simulink model "DynamicModelComplete"  (R2022b)
settings: configuration reference "WheelSimConfiguration" (kept outside this file)
settings Model: Creator=At  LastModifiedBy=MOSA
settings ConfigSetRef: SourceName=WheelSimConfiguration  SourceLocation=Base Workspace

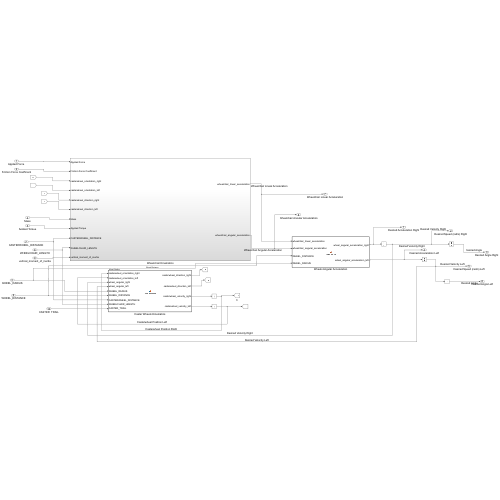
[thumbnail: Simulink's stored preview of the top-level diagram]
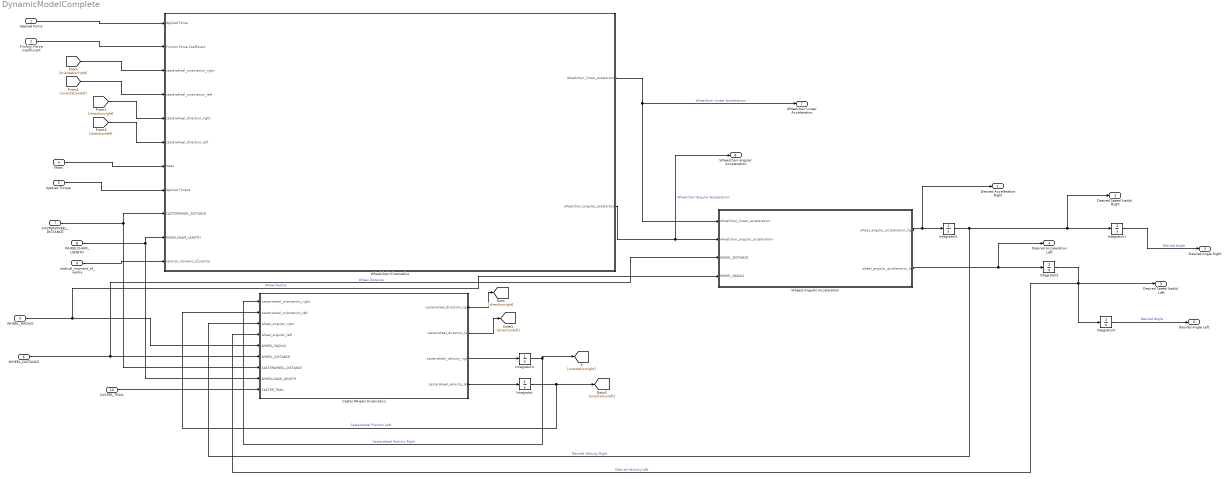
== system DynamicModelComplete ==
  "Applied Force " : Inport
  Friction Force Coefficient : Inport  Port=2
  WHEEL_RADIUS : Inport  Port=3
  Mass : Inport  Port=4
  Applied Torque : Inport  Port=5
  WHEEL_DISTANCE : Inport  Port=6
  CASTERWHEEL_DISTANCE : Inport  Port=7
  WHEELCHAIR_LENGTH : Inport  Port=8
  vertical_moment_of_inertia : Inport  Port=9
  CASTER_TRAIL : Inport  Port=10
  Caster Wheels Kinematics : MATLAB Function  TreatAsAtomicUnit=on
  Integrator{,1..5} (6 alike) : Integrator
  Wheelchair Kinematics : Subsystem
  Wheels Angular Acceleration : MATLAB Function  TreatAsAtomicUnit=on
  Desired Acceleration Right : Outport
  Desired Speed (rad/s) Right : Outport  Port=2
  Desired Angle Right : Outport  Port=3
  Desired Acceleration Left : Outport  Port=4
  Desired Speed (rad/s) Left : Outport  Port=5
  Desired Angle Left : Outport  Port=6
  Wheelchair Linear Acceleration : Outport  Port=7
  Wheelchair Angular Acceleration : Outport  Port=8
  wires:
  Integrator5/1 -> Caster Wheels Kinematics/3(wheel_angular_right), Integrator1/1, Desired Speed (rad/s) Right/1  "Desired Velocity Right"
  Integrator1/1 -> Desired Angle Right/1  "Desired Angle"
  Integrator2/1 -> Caster Wheels Kinematics/4(wheel_angular_left), Desired Speed (rad/s) Left/1, Integrator3/1  "Desired Velocity Left"
  Integrator3/1 -> Desired Angle Left/1  "Desired Angle"
  Wheels Angular Acceleration/1(wheel_angular_acceleration_right) -> Desired Acceleration Right/1, Integrator5/1
  Wheelchair Kinematics/1(wheelchair_linear_acceleration) -> Wheels Angular Acceleration/1(wheelchair_linear_acceleration), Wheelchair Linear Acceleration/1  "Wheelchair Linear Acceleration"
  Wheelchair Kinematics/2(wheelchair_angular_acceleration) -> Wheelchair Angular Acceleration/1, Wheels Angular Acceleration/2(wheelchair_angular_acceleration)  "Wheelchair Angular Acceleration"
  CASTERWHEEL_DISTANCE/1 -> Caster Wheels Kinematics/7(CASTERWHEEL_DISTANCE), Wheelchair Kinematics/9(CASTERWHEEL_DISTANCE)
  WHEELCHAIR_LENGTH/1 -> Caster Wheels Kinematics/8(WHEELCHAIR_LENGTH), Wheelchair Kinematics/10(WHEELCHAIR_LENGTH)
  vertical_moment_of_inertia/1 -> Wheelchair Kinematics/11(vertical_moment_of_inertia)
  "Applied Force "/1 -> Wheelchair Kinematics/1("Applied Force ")
  Friction Force Coefficient/1 -> Wheelchair Kinematics/2(Friction Force Coefficient)
  Mass/1 -> Wheelchair Kinematics/7(Mass)
  Applied Torque/1 -> Wheelchair Kinematics/8(Applied Torque)
  Caster Wheels Kinematics/3(casterwheel_velocity_right) -> Integrator4/1
  Caster Wheels Kinematics/4(casterwheel_velocity_left) -> Integrator/1
  Caster Wheels Kinematics/1(casterwheel_direction_right) -> [directionright]
  Integrator/1 -> [orientationleft], Caster Wheels Kinematics/2(casterwheel_orientation_left)  "Casterwheel Position Left"
  Integrator4/1 -> [orientationright], Caster Wheels Kinematics/1(casterwheel_orientation_right)  "Casterwheel Position Right"
  Caster Wheels Kinematics/2(casterwheel_direction_left) -> [directionleft]
  [directionleft] -> Wheelchair Kinematics/6(casterwheel_direction_left)
  [directionright] -> Wheelchair Kinematics/5(casterwheel_direction_right)
  [orientationleft] -> Wheelchair Kinematics/4(casterwheel_orientation_left)
  [orientationright] -> Wheelchair Kinematics/3(casterwheel_orientation_right)
  Wheels Angular Acceleration/2(wheel_angular_acceleration_left) -> Desired Acceleration Left/1, Integrator2/1
  CASTER_TRAIL/1 -> Caster Wheels Kinematics/9(CASTER_TRAIL)
  WHEEL_RADIUS/1 -> Wheels Angular Acceleration/4(WHEEL_RADIUS), Caster Wheels Kinematics/5(WHEEL_RADIUS)  "Wheel Radius"
  WHEEL_DISTANCE/1 -> Wheels Angular Acceleration/3(WHEEL_DISTANCE), Caster Wheels Kinematics/6(WHEEL_DISTANCE)  "Wheel Distance"

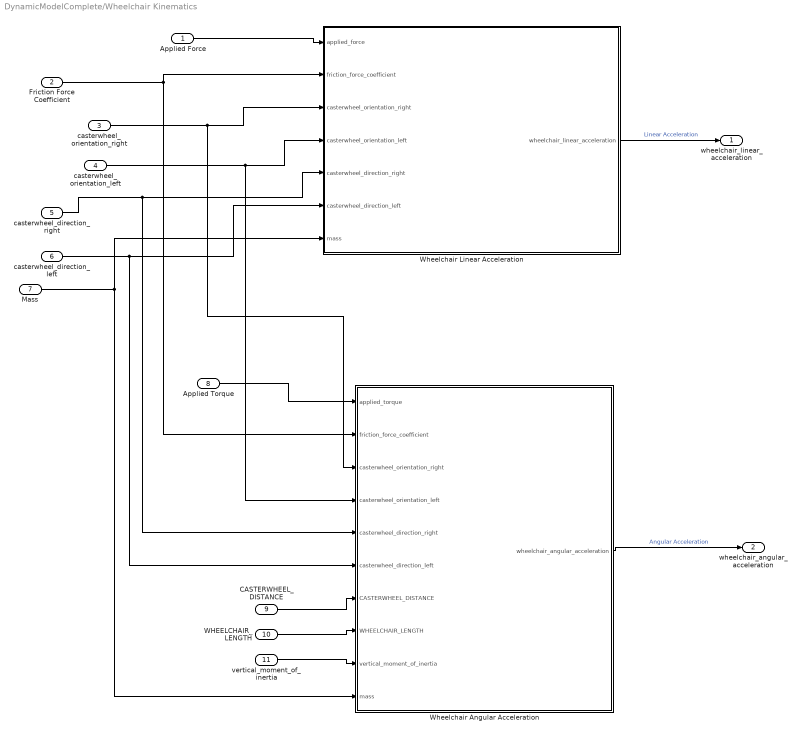
== system DynamicModelComplete/Wheelchair Kinematics ==
  "Applied Force " : Inport
  Friction Force Coefficient : Inport  Port=2
  casterwheel_orientation_right : Inport  Port=3
  casterwheel_orientation_left : Inport  Port=4
  casterwheel_direction_right : Inport  Port=5
  casterwheel_direction_left : Inport  Port=6
  Mass : Inport  Port=7
  Applied Torque : Inport  Port=8
  CASTERWHEEL_DISTANCE : Inport  Port=9
  WHEELCHAIR_LENGTH : Inport  Port=10
  vertical_moment_of_inertia : Inport  Port=11
  Wheelchair Angular Acceleration : MATLAB Function  TreatAsAtomicUnit=on
  Wheelchair Linear Acceleration : MATLAB Function  TreatAsAtomicUnit=on
  wheelchair_linear_acceleration : Outport
  wheelchair_angular_acceleration : Outport  Port=2
  wires:
  "Applied Force "/1 -> Wheelchair Linear Acceleration/1(applied_force)
  Mass/1 -> Wheelchair Angular Acceleration/10(mass), Wheelchair Linear Acceleration/7(mass)
  Applied Torque/1 -> Wheelchair Angular Acceleration/1(applied_torque)
  Wheelchair Linear Acceleration/1(wheelchair_linear_acceleration) -> wheelchair_linear_acceleration/1  "Linear Acceleration"
  Wheelchair Angular Acceleration/1(wheelchair_angular_acceleration) -> wheelchair_angular_acceleration/1  "Angular Acceleration"
  Friction Force Coefficient/1 -> Wheelchair Angular Acceleration/2(friction_force_coefficient), Wheelchair Linear Acceleration/2(friction_force_coefficient)
  casterwheel_orientation_right/1 -> Wheelchair Angular Acceleration/3(casterwheel_orientation_right), Wheelchair Linear Acceleration/3(casterwheel_orientation_right)
  casterwheel_orientation_left/1 -> Wheelchair Angular Acceleration/4(casterwheel_orientation_left), Wheelchair Linear Acceleration/4(casterwheel_orientation_left)
  casterwheel_direction_right/1 -> Wheelchair Angular Acceleration/5(casterwheel_direction_right), Wheelchair Linear Acceleration/5(casterwheel_direction_right)
  casterwheel_direction_left/1 -> Wheelchair Angular Acceleration/6(casterwheel_direction_left), Wheelchair Linear Acceleration/6(casterwheel_direction_left)
  CASTERWHEEL_DISTANCE/1 -> Wheelchair Angular Acceleration/7(CASTERWHEEL_DISTANCE)
  WHEELCHAIR_LENGTH/1 -> Wheelchair Angular Acceleration/8(WHEELCHAIR_LENGTH)
  vertical_moment_of_inertia/1 -> Wheelchair Angular Acceleration/9(vertical_moment_of_inertia)

== matlab function DynamicModelComplete/Wheelchair Kinematics/Wheelchair Angular Acceleration ==
  data: applied_torque input; friction_force_coefficient input; casterwheel_orientation_right input; casterwheel_orientation_left input; casterwheel_direction_right input; casterwheel_direction_left input; CASTERWHEEL_DISTANCE input; WHEELCHAIR_LENGTH input; vertical_moment_of_inertia input; wheelchair_angular_acceleration output; mass input
function wheelchair_angular_acceleration  = wheelchair_angular(applied_torque, friction_force_coefficient, casterwheel_orientation_right,...
casterwheel_orientation_left, casterwheel_direction_right,casterwheel_direction_left,...
CASTERWHEEL_DISTANCE,WHEELCHAIR_LENGTH,vertical_moment_of_inertia,mass)

%% This function calculates the wheelchair angular acceleration based on the information from casterwheel estimator
g=9.81;

friction_force=friction_force_coefficient*mass*g;

sum_of_torques = (applied_torque + ((friction_force * CASTERWHEEL_DISTANCE/4)*...
    (casterwheel_direction_left*cos(casterwheel_orientation_left)-casterwheel_direction_right*cos(casterwheel_orientation_right)))-...
    ((friction_force *WHEELCHAIR_LENGTH/2)*...
    (casterwheel_direction_left*sin(casterwheel_orientation_left)+casterwheel_direction_right*sin(casterwheel_orientation_right)))) ;

wheelchair_angular_acceleration = sum_of_torques / (vertical_moment_of_inertia);

== matlab function DynamicModelComplete/Wheelchair Kinematics/Wheelchair Linear Acceleration ==
  data: applied_force input; friction_force_coefficient input; casterwheel_orientation_right input; casterwheel_orientation_left input; casterwheel_direction_right input; casterwheel_direction_left input; wheelchair_linear_acceleration output; mass input
function wheelchair_linear_acceleration  = wheelchair_linear(applied_force, friction_force_coefficient, casterwheel_orientation_right,...
casterwheel_orientation_left, casterwheel_direction_right,casterwheel_direction_left, mass)

%% This function calculates the wheelchair linear acceleration based on the information from casterwheel estimator
g=9.81;

friction_force=friction_force_coefficient*mass*g;

sum_of_forces = (applied_force - (friction_force * ...
    (casterwheel_direction_right*cos(casterwheel_orientation_right)+casterwheel_direction_left*cos(casterwheel_orientation_left))/ 2)) ;

wheelchair_linear_acceleration = sum_of_forces / mass;

== matlab function DynamicModelComplete/Wheels Angular Acceleration ==
  data: wheelchair_linear_acceleration input; wheel_angular_acceleration_right output; wheelchair_angular_acceleration input; wheel_angular_acceleration_left output; WHEEL_DISTANCE input; WHEEL_RADIUS input
function [wheel_angular_acceleration_right,wheel_angular_acceleration_left] =...
    wheel_angular(wheelchair_linear_acceleration,wheelchair_angular_acceleration,WHEEL_DISTANCE,WHEEL_RADIUS)
%% This function calculates  wheels' acceleration based on the linear and angular acceleration of wheelchair




wheel_angular_acceleration_right=wheelchair_linear_acceleration/WHEEL_RADIUS+wheelchair_angular_acceleration*(WHEEL_DISTANCE/(2*WHEEL_RADIUS));
wheel_angular_acceleration_left=wheelchair_linear_acceleration/WHEEL_RADIUS-wheelchair_angular_acceleration*(WHEEL_DISTANCE/(2*WHEEL_RADIUS));

== matlab function DynamicModelComplete/Caster Wheels Kinematics ==
  data: casterwheel_orientation_right input; casterwheel_orientation_left input; wheel_angular_right input; wheel_angular_left input; WHEEL_RADIUS input; WHEEL_DISTANCE input; CASTERWHEEL_DISTANCE input; WHEELCHAIR_LENGTH input; CASTER_TRAIL input; casterwheel_direction_right output; casterwheel_direction_left output; casterwheel_velocity_right output; casterwheel_velocity_left output
function [casterwheel_direction_right,casterwheel_direction_left, casterwheel_velocity_right,casterwheel_velocity_left]  =...
    caster_kinematics(casterwheel_orientation_right,casterwheel_orientation_left,...
wheel_angular_right,wheel_angular_left,WHEEL_RADIUS,WHEEL_DISTANCE,CASTERWHEEL_DISTANCE,WHEELCHAIR_LENGTH,...
CASTER_TRAIL)

%% This function is the casterwheel estimator

casterwheel_velocity_right=(WHEEL_RADIUS*(wheel_angular_right-wheel_angular_left)/(CASTER_TRAIL*WHEEL_DISTANCE))*...
    (WHEELCHAIR_LENGTH*cos(casterwheel_orientation_right)-(CASTERWHEEL_DISTANCE*sin(casterwheel_orientation_right)/2)-CASTER_TRAIL)-...
    (WHEEL_RADIUS*((wheel_angular_right+wheel_angular_left)/(2*CASTER_TRAIL))*sin(casterwheel_orientation_right));

casterwheel_velocity_left=(WHEEL_RADIUS*(wheel_angular_right-wheel_angular_left)/(CASTER_TRAIL*WHEEL_DISTANCE))*...
    (WHEELCHAIR_LENGTH*cos(casterwheel_orientation_left)+(CASTERWHEEL_DISTANCE*sin(casterwheel_orientation_left)/2)-CASTER_TRAIL)-...
    (WHEEL_RADIUS*((wheel_angular_right+wheel_angular_left)/(2*CASTER_TRAIL))*sin(casterwheel_orientation_left));

casterwheel_direction_right=sign((WHEEL_RADIUS*((wheel_angular_right+wheel_angular_left)/2)*cos(casterwheel_orientation_right)+...
    (WHEEL_RADIUS*((wheel_angular_right-wheel_angular_left)/WHEEL_DISTANCE)*...
    (WHEELCHAIR_LENGTH*sin(casterwheel_orientation_right)+((CASTERWHEEL_DISTANCE/2)*cos(casterwheel_orientation_right))))));

casterwheel_direction_left=sign((WHEEL_RADIUS*((wheel_angular_right+wheel_angular_left)/2)*cos(casterwheel_orientation_left)+...
    (WHEEL_RADIUS*((wheel_angular_right-wheel_angular_left)/WHEEL_DISTANCE)*...
    (WHEELCHAIR_LENGTH*sin(casterwheel_orientation_left)-((CASTERWHEEL_DISTANCE/2)*cos(casterwheel_orientation_left))))));
